simulink model "Q1s"  (R2018a)
settings: Solver=VariableStepAuto  StartTime=0.0  StopTime=100  RelTol=1e-3
settings Model: Creator=Halil Temurtaş  LastModifiedBy=Halil Temurtaş

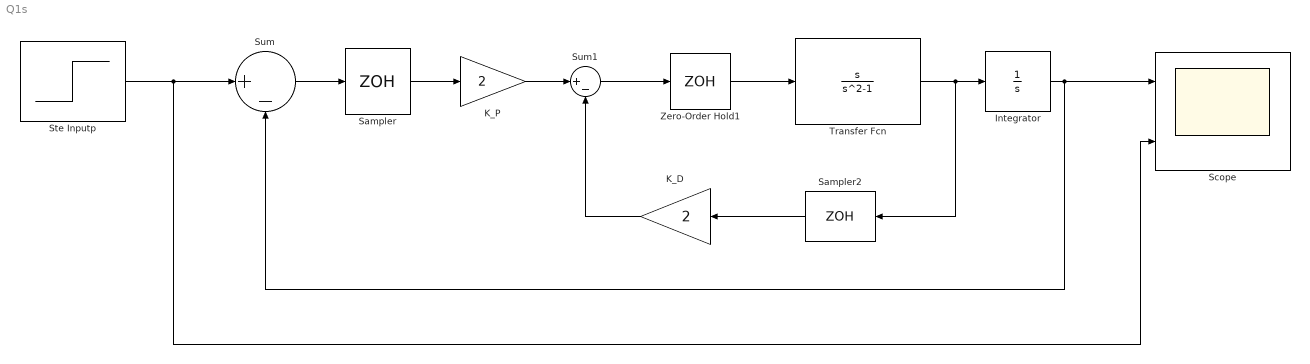
== system Q1s ==
  Integrator : Integrator
  K_D : Gain  Gain=2
  K_P : Gain  Gain=2
  Sampler : ZeroOrderHold  SampleTime=-1
  Sampler2 : ZeroOrderHold  SampleTime=-1
  Scope : Scope  NumInputPorts=2
  Ste Inputp : Step  Time=0  SampleTime=0
  Sum : Sum  Inputs=|+-
  Sum1 : Sum  Inputs=|+-
  Transfer Fcn : TransferFcn  Numerator=[1 0]  Denominator=[1 0 -1]
  Zero-Order Hold1 : ZeroOrderHold  SampleTime=-1
  wires:
  Integrator/1 -> Scope/1, Sum/2
  Sampler/1 -> K_P/1
  Zero-Order Hold1/1 -> Transfer Fcn/1
  Transfer Fcn/1 -> Sampler2/1, Integrator/1
  Ste Inputp/1 -> Scope/2, Sum/1
  Sum/1 -> Sampler/1
  Sum1/1 -> Zero-Order Hold1/1
  K_P/1 -> Sum1/1
  K_D/1 -> Sum1/2
  Sampler2/1 -> K_D/1
